simulink model "WPT_varyingU"  (R2022b)
settings: Solver=VariableStepAuto  StartTime=0.0  StopTime=10.0  RelTol=1e-3
undefined symbols (not defined in the file): plecs
settings Model: Creator=dcostine  LastModifiedBy=dcostine
settings DebuggingCC: UnconnectedInputMsg=warning  UnconnectedOutputMsg=warning  UnconnectedLineMsg=warning
settings ModelReferenceCC: EnableRefExpFcnMdlSchedulingChecks=on
settings RTWCC: DLArmComputeVersion=19.05

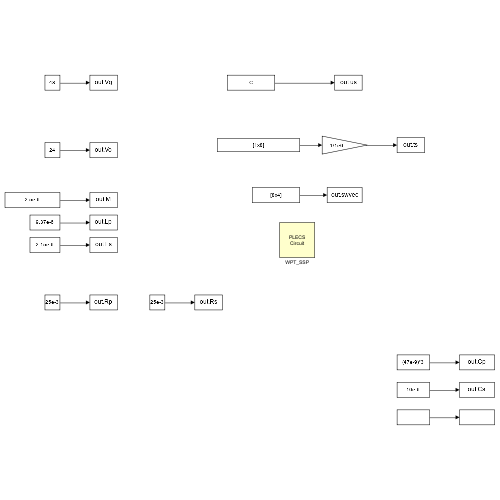
[thumbnail: Simulink's stored preview of the top-level diagram]
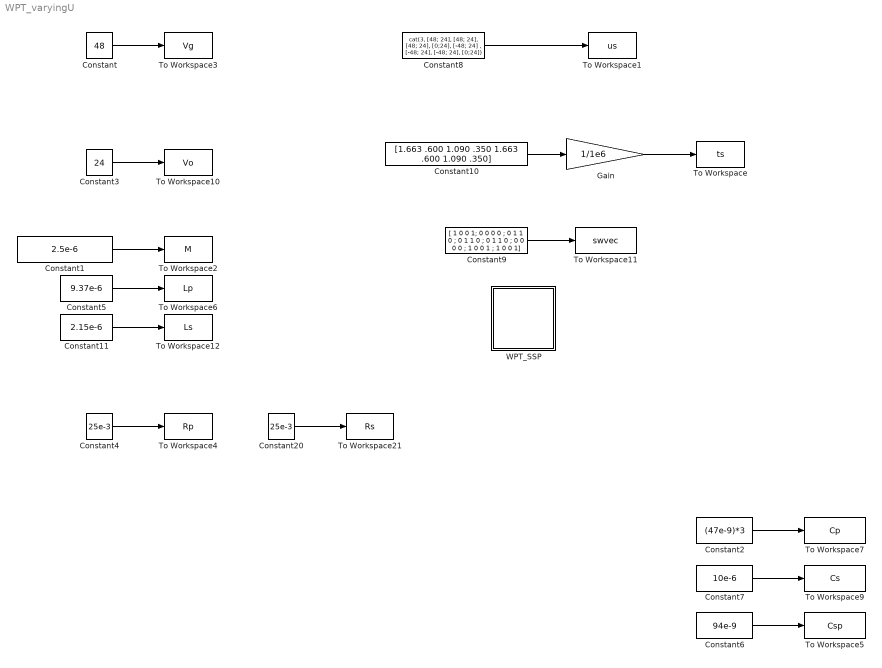
== system WPT_varyingU ==
  Constant : Constant  Value=48
  Constant1 : Constant  Value=2.5e-6
  Constant10 : Constant  Value="[1.663 .600  1.090 .350 1.663 .600  1.090 .350]"
  Constant11 : Constant  Value=2.15e-6
  Constant2 : Constant  Value=(47e-9)*3
  Constant20 : Constant  Value=25e-3
  Constant3 : Constant  Value=24
  Constant4 : Constant  Value=25e-3
  Constant5 : Constant  Value=9.37e-6
  Constant6 : Constant  Value=94e-9
  Constant7 : Constant  Value=10e-6
  Constant8 : Constant  Value=cat(3, [48; 24], [48; 24], [48; 24], [0;24], [-48; 24] , [-48; 24], [-48; 24], [0;24])
  Constant9 : Constant  Value=|
      | [ 1     0     0     1;
      |      0     0     0     0
      | ;     0     1     1     0
      | ;     0     1     1     0
      | ;     0     1     1     0
      |  ;    0     0     0     0
      |  ;    1     0     0     1
      |  ;    1     0     0     1]
  Gain : Gain  Gain=1/1e6
  To Workspace : ToWorkspace  VariableName=ts  SampleTime=-1
  To Workspace1 : ToWorkspace  VariableName=us  SampleTime=-1
  To Workspace10 : ToWorkspace  VariableName=Vo  SampleTime=-1
  To Workspace11 : ToWorkspace  VariableName=swvec  SampleTime=-1
  To Workspace12 : ToWorkspace  VariableName=Ls  SampleTime=-1
  To Workspace2 : ToWorkspace  VariableName=M  SampleTime=-1
  To Workspace21 : ToWorkspace  VariableName=Rs  SampleTime=-1
  To Workspace3 : ToWorkspace  VariableName=Vg  SampleTime=-1
  To Workspace4 : ToWorkspace  VariableName=Rp  SampleTime=-1
  To Workspace5 : ToWorkspace  VariableName=Csp  SampleTime=-1
  To Workspace6 : ToWorkspace  VariableName=Lp  SampleTime=-1
  To Workspace7 : ToWorkspace  VariableName=Cp  SampleTime=-1
  To Workspace9 : ToWorkspace  VariableName=Cs  SampleTime=-1
  WPT_SSP : Subsystem  LoadFcn=plecs('sl', 200);  InitFcn=plecs('sl', 214);  StartFcn=plecs('sl', 208);  StopFcn=plecs('sl', 209);  mask(PlecsCircuit){PLECSData=<binary blob, 2128 chars, not shown>}
      mask prompts: PLECSData "PLECS Data (Do not delete or modify!)"
      mask init:
      | % PLACE CUSTOM INITIALIZATIONS ABOVE
      | % DO NOT REMOVE
      | plecs('sl', 215);
      | % DO NOT REMOVE
      settings: CopyFcn=plecs('sl', 203);  DeleteFcn=plecs('sl', 205);  UndoDeleteFcn=plecs('sl', 206);  PreSaveFcn=plecs('sl', 211);  PostSaveFcn=plecs('sl', 201);  NameChangeFcn=plecs('sl', 210);  DestroyFcn=plecs('sl', 207);  PreCopyFcn=plecs('sl', 216);  OpenFcn=plecs('sl', 202);  ErrorFcn=plerrorfcn
      mask Help: web(['file:///' fullfile(plecsdoc, 'creatingacircuit.html')])
      mask Display: disp('PLECS\nCircuit')
  wires:
  Constant5/1 -> To Workspace6/1
  Constant/1 -> To Workspace3/1
  Constant3/1 -> To Workspace10/1
  Constant1/1 -> To Workspace2/1
  Constant4/1 -> To Workspace4/1
  Constant20/1 -> To Workspace21/1
  Constant2/1 -> To Workspace7/1
  Constant7/1 -> To Workspace9/1
  Constant11/1 -> To Workspace12/1
  Constant6/1 -> To Workspace5/1
  Constant10/1 -> Gain/1
  Constant9/1 -> To Workspace11/1
  Gain/1 -> To Workspace/1
  Constant8/1 -> To Workspace1/1

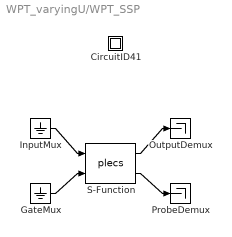
== system WPT_varyingU/WPT_SSP ==
  " CircuitID41 " : Subsystem
  " GateMux " : Ground
  " InputMux " : Ground
  " OutputDemux " : Terminator
  " ProbeDemux " : Terminator
  " S-Function " : S-Function  FunctionName=plecs  SFunctionDeploymentMode=off  EnableBusSupport=off
  wires:
  " InputMux "/1 -> " S-Function "/1
  " GateMux "/1 -> " S-Function "/2
  " S-Function "/1 -> " OutputDemux "/1
  " S-Function "/2 -> " ProbeDemux "/1

== system WPT_varyingU/WPT_SSP/ CircuitID41  ==
